simulink model "washing_machine"  (R2024b)
settings: Solver=VariableStepAuto  StartTime=0.0  StopTime=70  RelTol=1e-3
settings Model: Creator=Admin  LastModifiedBy=Admin

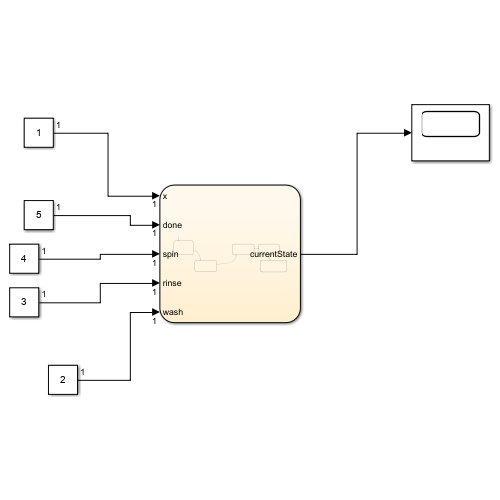
[thumbnail: Simulink's stored preview of the top-level diagram]
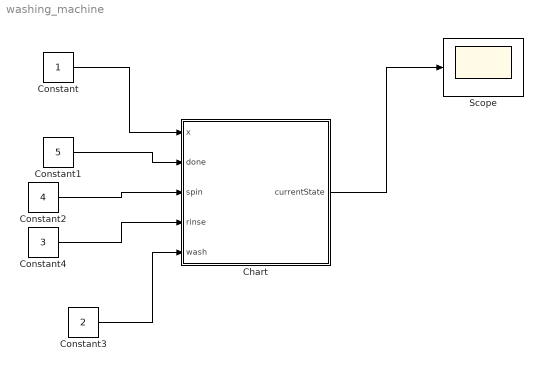
== system washing_machine ==
  Chart : Stateflow chart  TreatAsAtomicUnit=on
  Constant : Constant
  Constant1 : Constant  Value=5
  Constant2 : Constant  Value=4
  Constant3 : Constant  Value=2
  Constant4 : Constant  Value=3
  Scope : Scope
  wires:
  Chart/1(currentState) -> Scope/1
  Constant/1 -> Chart/1(x)
  Constant1/1 -> Chart/2(done)
  Constant2/1 -> Chart/3(spin)
  Constant4/1 -> Chart/4(rinse)
  Constant3/1 -> Chart/5(wash)

== stateflow chart washing_machine/Chart ==
  state fill
    entry:
    x=1;
    currentState = fill;
    disp("Filling water...")
  state rinse
    entry:
    x=3;
    currentState = rinse;
    disp("Rinsing clothes...")
  state spin
    entry:
    x=4;
    currentState = spin;
    disp("Spinning clothes...")
  state done
    entry:
    x=5;
    currentState = done;
    disp("Washing cycle complete.")
  state wash
    entry:
    x=2;
    currentState = wash;
    disp("Washing clothes...")
  (default) -> fill
  rinse -> spin : after(15,sec)
  fill -> wash : after(10,sec)
  wash -> rinse : after(20,sec)
  spin -> done : after(10,sec)
  data: x input; currentState output; done input; spin input; rinse input; wash input
